simulink model "rectifythreephase"  (Simulink 7.8)
settings: Solver=ode45  StartTime=0.0  StopTime=0.1  RelTol=1e-3
libraries: powerlib x12, powerlib_extras x1
settings Model: Creator=Administrator  LastModifiedBy=赵
settings DebuggingCC: FcnCallInpInsideContextMsg=Use local settings  StrictBusMsg=Warning

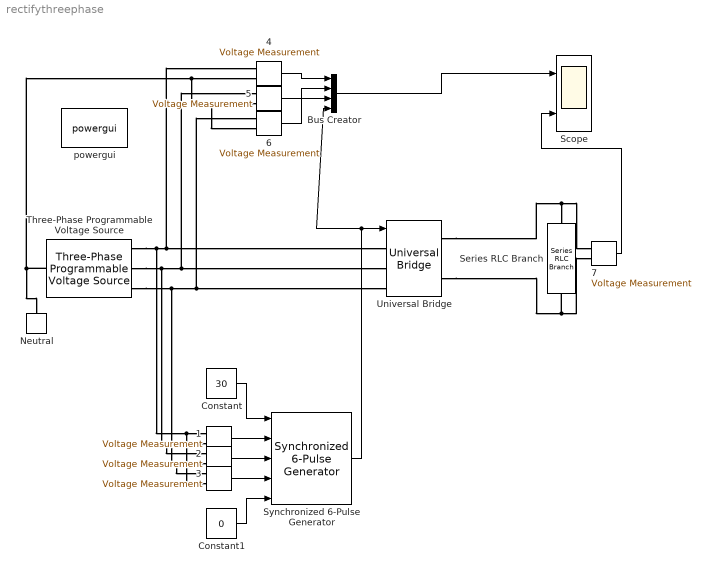
== system rectifythreephase ==
  {1..7} (7 alike) : powerlib/Measurements/Voltage Measurement  PhasorSimulation=off  OutputType=Complex  PSBequivalent=0
  Bus Creator : BusCreator
  Constant : Constant  Value=30
  Constant1 : Constant  Value=0
  Neutral : powerlib/Elements/Neutral  LConnTagsString=a  NodeNumber=10
  Scope : Scope  NumInputPorts=2
      settings: YMin=-5~-5  YMax=5~5
  Series RLC Branch : powerlib/Elements/Series RLC Branch  LConnTagsString=__new0  RConnTagsString=__new0  BranchType=R  Resistance=2  Inductance=1  SetiL0=off  InitialCurrent=0  Capacitance=1e-6  Setx0=off  InitialVoltage=0  Measurements=None
  Synchronized 6-Pulse Generator : powerlib_extras/Control  Blocks/Synchronized 6-Pulse Generator  freq=50  pwidth=10  Double_Pulse=off
  Three-Phase Programmable Voltage Source : powerlib/Electrical Sources/Three-Phase Programmable Voltage Source  PositiveSequence="[100  0 50]"  VariationEntity=None  VariationType=Step  VariationStep=0.5  VariationRate=10  VariationMagnitude=0.3  VariationFrequency=2  VariationTiming=[1 2]  VariationPhaseA=off  Amplitudes=[1 0.8 1.2 1.0]  TimeValues=[0 0.1 0.15 0.2]  HarmonicGeneration=off  HarmonicA=[3 0.2 -25 0]  HarmonicB=[2 0.15 35 2]  Timing="[0.05  3]"  BusType=swing  Pref=0  Qref=0  Qmin=-inf  Qmax=inf
  Universal Bridge : powerlib/Power Electronics/Universal Bridge  Arms=3  SnubberResistance=1e5  SnubberCapacitance=inf  Device=Thyristors  Ron=1e-3  Lon=0  ForwardVoltages="[  0  0  ]"  ForwardVoltage=0  GTOparameters=[ 10e-6 , 20e-6 ]  IGBTparameters=[ 1e-6 , 2e-6 ]  Measurements=None  Measurements_2=None  converterType=Rectifier
  powergui : powerlib/powergui  Priority=1  SimulationMode=Continuous  SolverType=Tustin  SampleTime=50e-6  frequency=60  SPID=off  DisableSnubberDevices=off  DisableRonSwitches=off  DisableVfSwitches=off  SwTol=0  Interpol=off  DisplayEquations=off  FunctionMessages=off  frequencyindice=50  Pbase=100e6  ErrMax=1e-4  Iterations=50  UnitsV=kV  UnitsW=MW  echomessages=off  HookPort=off  EnableUseOfTLC=off  x0status=blocks  RestoreLinks=warning  ResistiveCurrentMeasurement=off  Frange=[0:2:500]  Ylog=off  Xlog=on  ShowGrid=off  save=off  variable=ZData  ZoomFFT=on  StartTime=0.0  cycles=1  DisplayStyle=1  fundamental=60  FreqAxis=off  MaxFrequency=1000  frequencyindicesteady=1  RmsSteady=1  display=off  Ts=0  methode=off
  wires:
  Synchronized 6-Pulse Generator/1 -> Universal Bridge/1, Bus Creator/4
  1/1 -> Synchronized 6-Pulse Generator/2
  2/1 -> Synchronized 6-Pulse Generator/3
  3/1 -> Synchronized 6-Pulse Generator/4
  Constant1/1 -> Synchronized 6-Pulse Generator/5
  Constant/1 -> Synchronized 6-Pulse Generator/1
  4/1 -> Bus Creator/1
  5/1 -> Bus Creator/2
  6/1 -> Bus Creator/3
  Bus Creator/1 -> Scope/1
  7/1 -> Scope/2
  connections:
  Universal Bridge/RConn1 -- Series RLC Branch/LConn1 -- 7/LConn1
  Universal Bridge/RConn2 -- Series RLC Branch/RConn1 -- 7/LConn2
  1/LConn1 -- 3/LConn2 -- Three-Phase Programmable Voltage Source/RConn1 -- Universal Bridge/LConn1 -- 4/LConn1
  1/LConn2 -- 2/LConn1 -- Three-Phase Programmable Voltage Source/RConn2 -- Universal Bridge/LConn2 -- 5/LConn1
  2/LConn2 -- 3/LConn1 -- Three-Phase Programmable Voltage Source/RConn3 -- Universal Bridge/LConn3 -- 6/LConn1
  Three-Phase Programmable Voltage Source/LConn1 -- Neutral/LConn1 -- 4/LConn2 -- 5/LConn2 -- 6/LConn2
